simulink model "control_project_compensated"  (R2016a)
settings: Solver=VariableStepAuto  StartTime=0.0  StopTime=10.0  RelTol=1e-3
settings Model: Creator=medo_  LastModifiedBy=medo_

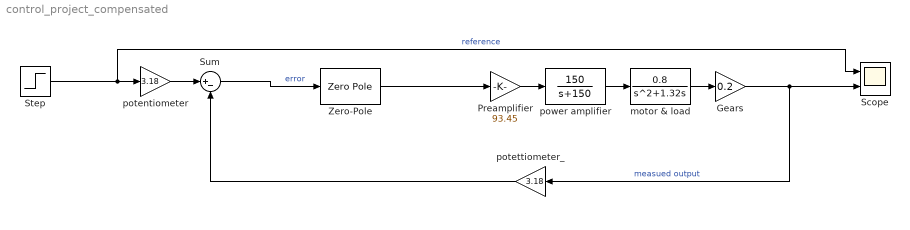
== system control_project_compensated ==
  Gears : Gain  Gain=0.2
  Preamplifier : Gain  Gain=93.45
  Scope : Scope  NumInputPorts=2
  Step : Step  SampleTime=0
  Sum : Sum  Inputs=|+-
  Zero-Pole : ZeroPole  Zeros=[-2 -0.01]  Poles=[0 -150 -1.32 -3.708 -0.001]  Gain=[1434.053]
  motor & load : TransferFcn  Numerator=[0.8]  Denominator=[1 1.32 0]
  potentiometer : Gain  Gain=3.18
  potettiometer_ : Gain  Gain=3.18
  power amplifier : TransferFcn  Numerator=[150]  Denominator=[1 150]
  wires:
  Gears/1 -> Scope/2, potettiometer_/1  "measued output"
  Sum/1 -> Zero-Pole/1  "error"
  ? -> ?  "control input"
  power amplifier/1 -> motor & load/1
  motor & load/1 -> Gears/1
  Preamplifier/1 -> power amplifier/1
  potentiometer/1 -> Sum/1
  Step/1 -> Scope/1, potentiometer/1  "reference"
  potettiometer_/1 -> Sum/2
  Zero-Pole/1 -> Preamplifier/1
